simulink model "SolderingIronPIDControllerV2"  (R2024b)
settings: Solver=VariableStepAuto  StartTime=0.0  StopTime=200  RelTol=1e-3
libraries: slpidlib x1
settings Model: Creator=ken  LastModifiedBy=ken

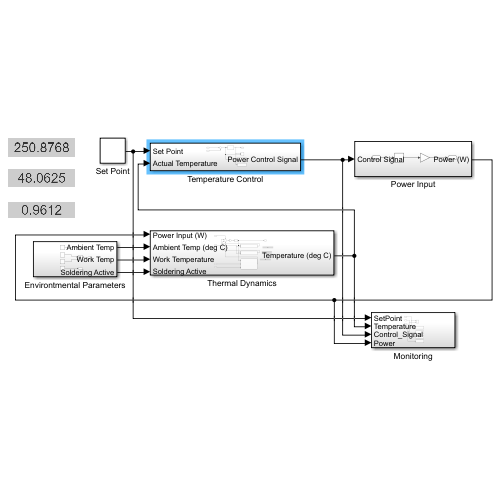
[thumbnail: Simulink's stored preview of the top-level diagram]
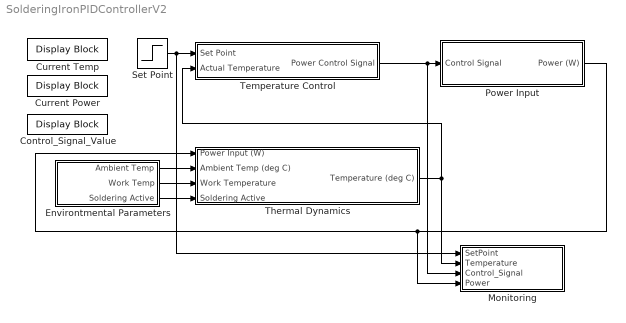
== system SolderingIronPIDControllerV2 ==
  Control_Signal_Value : DisplayBlock  LabelPosition=Hide  Transparency=1
  Current Power : DisplayBlock  LabelPosition=Hide  Transparency=1
  Current Temp : DisplayBlock  LabelPosition=Hide  Transparency=1
  Environtmental Parameters : Subsystem
  Monitoring : Subsystem
  Power Input : Subsystem
  Set Point : Step  Before=250  After=250  SampleTime=0
  Temperature Control : Subsystem
  Thermal Dynamics : Subsystem
  wires:
  Set Point/1 -> Temperature Control/1(Set Point), Monitoring/1(SetPoint)
  Thermal Dynamics/1(Temperature (deg C)) -> Monitoring/2(Temperature), Temperature Control/2(Actual Temperature)
  Temperature Control/1(Power Control Signal) -> Monitoring/3(Control_Signal), Power Input/1(Control Signal)
  Power Input/1(Power (W)) -> Monitoring/4(Power), Thermal Dynamics/1(Power Input (W))
  Environtmental Parameters/1(Ambient Temp) -> Thermal Dynamics/2(Ambient Temp (deg C))
  Environtmental Parameters/2(Work Temp) -> Thermal Dynamics/3(Work Temperature)
  Environtmental Parameters/3(Soldering Active) -> Thermal Dynamics/4(Soldering Active)

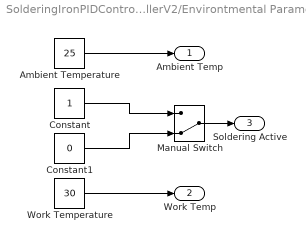
== system SolderingIronPIDControllerV2/Environtmental Parameters ==
  Ambient Temperature : Constant  Value=25
  Constant : Constant
  Constant1 : Constant  Value=0
  Manual Switch : ManualSwitch  CurrentSetting=0
  Work Temperature : Constant  Value=30
  Ambient Temp : Outport
  Work Temp : Outport  Port=2
  Soldering Active : Outport  Port=3
  wires:
  Ambient Temperature/1 -> Ambient Temp/1
  Work Temperature/1 -> Work Temp/1
  Constant/1 -> Manual Switch/1
  Constant1/1 -> Manual Switch/2
  Manual Switch/1 -> Soldering Active/1

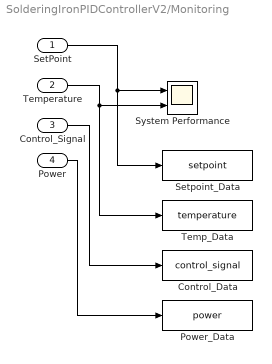
== system SolderingIronPIDControllerV2/Monitoring ==
  SetPoint : Inport
  Temperature : Inport  Port=2
  Control_Signal : Inport  Port=3
  Power : Inport  Port=4
  Control_Data : ToWorkspace  VariableName=control_signal  SaveFormat=Structure With Time  SampleTime=-1
  Power_Data : ToWorkspace  VariableName=power  SaveFormat=Structure With Time  SampleTime=-1
  Setpoint_Data : ToWorkspace  VariableName=setpoint  SaveFormat=Structure With Time  SampleTime=-1
  System Performance : Scope  NumInputPorts=2
  Temp_Data : ToWorkspace  VariableName=temperature  SaveFormat=Structure With Time  SampleTime=-1
  wires:
  SetPoint/1 -> System Performance/1, Setpoint_Data/1
  Temperature/1 -> System Performance/2, Temp_Data/1
  Control_Signal/1 -> Control_Data/1
  Power/1 -> Power_Data/1

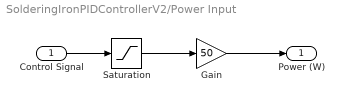
== system SolderingIronPIDControllerV2/Power Input ==
  Control Signal : Inport
  Gain : Gain  Gain=50  OutMax=60
  Saturation : Saturate  UpperLimit=1  LowerLimit=0
  Power (W) : Outport
  wires:
  Control Signal/1 -> Saturation/1
  Saturation/1 -> Gain/1
  Gain/1 -> Power (W)/1

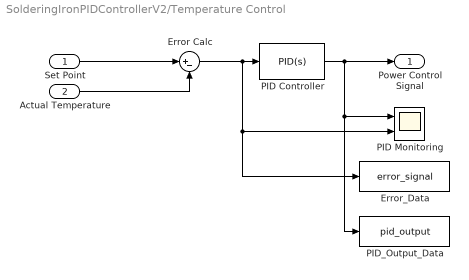
== system SolderingIronPIDControllerV2/Temperature Control ==
  Set Point : Inport
  Actual Temperature : Inport  Port=2
  Error Calc : Sum  Inputs=|+-
  Error_Data : ToWorkspace  VariableName=error_signal  SaveFormat=Structure With Time  SampleTime=-1
  PID Controller : slpidlib/PID Controller  Controller=PID  Form=Parallel  TimeDomain=Continuous-time  UseExternalTs=off  SampleTime=-1  IntegratorMethod=Forward Euler  FilterMethod=Forward Euler  ControllerParametersSource=internal  P=6  I=0.001  UseKiTs=off  D=0.001  UseExternalDerivativeSource=off  N=100  UseFilter=on  TunerSelectOption=Transfer Function Based (PID Tuner App)  InitialConditionSource=internal  InitialConditionForIntegrator=0  InitialConditionForFilter=0  DifferentiatorICPrevScaledInput=0  ExternalReset=none  TrackingMode=off  Kt=1  LimitOutput=on  SatLimitsSource=internal  UpperSaturationLimit=1  LowerSaturationLimit=0  LinearizeAsGain=on  AntiWindupMode=none  Kb=1  LimitIntegrator=off  UpperIntegratorSaturationLimit=inf  LowerIntegratorSaturationLimit=-inf  POutMin=[]  POutMax=[]  IOutMin=[]  IOutMax=[]  DOutMin=[]  DOutMax=[]  NOutMin=[]  NOutMax=[]  SumOutMin=[]  SumOutMax=[]  SaturationOutMin=[]  SaturationOutMax=[]  PParamMin=[]  PParamMax=[]  IParamMin=[]  IParamMax=[]  DParamMin=[]  DParamMax=[]  NParamMin=[]  NParamMax=[]  KbParamMin=[]  KbParamMax=[]  KtParamMin=[]  KtParamMax=[]  KbOutMin=[]  KbOutMax=[]  KtOutMin=[]  KtOutMax=[]  IntegratorOutMin=[]  IntegratorOutMax=[]  FilterOutMin=[]  FilterOutMax=[]  SumI1OutMin=[]  SumI1OutMax=[]  SumI2OutMin=[]  SumI2OutMax=[]  SumI3OutMin=[]  SumI3OutMax=[]  SumI4OutMin=[]  SumI4OutMax=[]  SumDOutMin=[]  SumDOutMax=[]  DifferentiatorOutMin=[]  DifferentiatorOutMax=[]  FilterDiffOutCoefMin=[]  FilterDiffOutCoefMax=[]  ReciprocalOutMin=[]  ReciprocalOutMax=[]  SumDenOutMin=[]  SumDenOutMax=[]  SumNumOutMin=[]  SumNumOutMax=[]  DivideOutMin=[]  DivideOutMax=[]  UdiffTsProdOutMin=[]  UdiffTsProdOutMax=[]  NTsProdOutMin=[]  NTsProdOutMax=[]  UintegralTsProdOutMin=[]  UintegralTsProdOutMax=[]  UngainTsProdOutMin=[]  UngainTsProdOutMax=[]  ClampingZeroOutDataTypeStr=Inherit: Inherit via back propagation  ClampingZeroOutMin=[]  ClampingZeroOutMax=[]  FilterDenConstantOutDataTypeStr=Inherit: Inherit via back propagation  FilterDenConstantOutMin=[]  FilterDenConstantOutMax=[]  PCopyOutDataTypeStr=Inherit: Inherit via back propagation  PCopyOutMin=[]  PCopyOutMax=[]  NCopyOutDataTypeStr=Inherit: Inherit via back propagation  NCopyOutMin=[]  NCopyOutMax=[]  IntegratorContinuousStateAttributes=''  IntegratorStateMustResolveToSignalObject=off  IntegratorRTWStateStorageClass=Auto  FilterContinuousStateAttributes=''  FilterStateMustResolveToSignalObject=off  FilterRTWStateStorageClass=Auto  ParallelPVariant=InternalParameters  IdealPVariant=Disabled  IVariant=InternalParameters  DVariant=InternalParameters  IntegratorVariant=Continuous  SatVariant=Enabled  AWVariant=Passthrough  PCopyVariant=Disabled  TRVariant=Disabled  FdbkBlocksVariant=Forward  IdealPFdbkVariant=Disabled  SatFdbkVariant=Disabled  DerivativeFilterVariant=ContFilter  NVariant=InternalParameters  NCopyVariant=Disabled  FilterICVariant=InternalICsFilter  IntegratorICVariant=InternalICs  ExternalResetVariant=Disabled  TRSumVariant=Passthrough  SumFdbkVariant=Disabled  SumVariant=Sum_PID  TsampFilterVariant=InternalTs  TsampNgainVariant=Passthrough  TsampIntegralVariant=Disabled_SignalSpec  ExternalSaturationOutDataTypeStr=Inherit: Same as second input  DerivativeSourceVariant=ErrorSignal  PreIntVariant=InternalPreInt
  PID Monitoring : Scope  NumInputPorts=2
  PID_Output_Data : ToWorkspace  VariableName=pid_output  SaveFormat=Structure With Time  SampleTime=-1
  Power Control Signal : Outport
  wires:
  Actual Temperature/1 -> Error Calc/2
  Error Calc/1 -> PID Controller/1, PID Monitoring/2, Error_Data/1
  PID Controller/1 -> PID Monitoring/1, PID_Output_Data/1, Power Control Signal/1
  Set Point/1 -> Error Calc/1

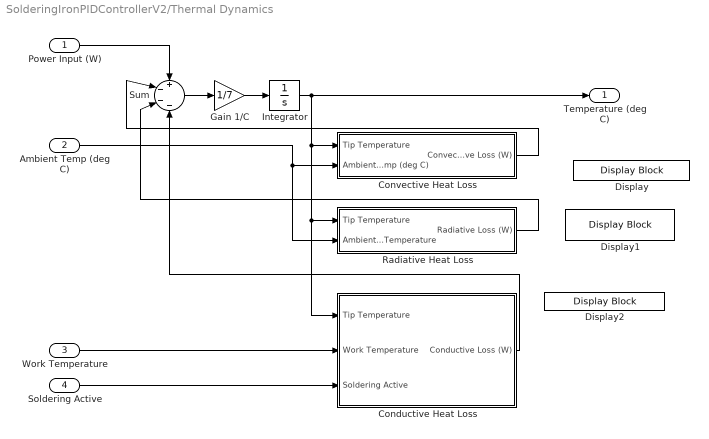
== system SolderingIronPIDControllerV2/Thermal Dynamics ==
  Power Input (W) : Inport
  Ambient Temp (deg C) : Inport  Port=2
  Work Temperature : Inport  Port=3
  Soldering Active : Inport  Port=4
  Conductive Heat Loss : Subsystem
  Convective Heat Loss : Subsystem
  Display : DisplayBlock  LabelPosition=Hide  Transparency=1
  Display1 : DisplayBlock  LabelPosition=Hide  Transparency=1
  Display2 : DisplayBlock  LabelPosition=Hide  Transparency=1
  Gain 1/C : Gain  Gain=1/7
  Integrator : Integrator  InitialCondition=25  LimitOutput=on  UpperSaturationLimit=500  LowerSaturationLimit=25
  Radiative Heat Loss : Subsystem
  Sum : Sum  Inputs=+---
  Temperature (deg C) : Outport
  wires:
  Sum/1 -> Gain 1/C/1
  Gain 1/C/1 -> Integrator/1
  Integrator/1 -> Convective Heat Loss/1(Tip Temperature), Radiative Heat Loss/1(Tip Temperature), Conductive Heat Loss/1(Tip Temperature), Temperature (deg C)/1
  Ambient Temp (deg C)/1 -> Radiative Heat Loss/2(Ambient Temperature), Convective Heat Loss/2(Ambient Temp (deg C))
  Power Input (W)/1 -> Sum/1
  Convective Heat Loss/1(Convective Loss (W)) -> Sum/2
  Radiative Heat Loss/1(Radiative Loss (W)) -> Sum/3
  Conductive Heat Loss/1(Conductive Loss (W)) -> Sum/4
  Soldering Active/1 -> Conductive Heat Loss/3(Soldering Active)
  Work Temperature/1 -> Conductive Heat Loss/2(Work Temperature)

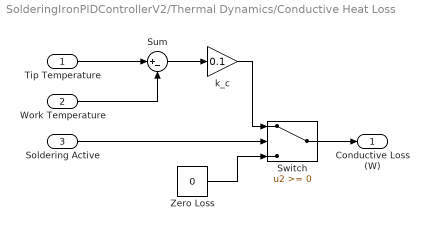
== system SolderingIronPIDControllerV2/Thermal Dynamics/Conductive Heat Loss ==
  Tip Temperature : Inport
  Work Temperature : Inport  Port=2
  Soldering Active : Inport  Port=3
  Sum : Sum  Inputs=|+-
  Switch : Switch  SaturateOnIntegerOverflow=off  InputSameDT=off
  Zero Loss : Constant  Value=0
  k_c : Gain  Gain=0.1
  Conductive Loss (W) : Outport
  wires:
  Tip Temperature/1 -> Sum/1
  Work Temperature/1 -> Sum/2
  Sum/1 -> k_c/1
  k_c/1 -> Switch/1
  Zero Loss/1 -> Switch/3
  Soldering Active/1 -> Switch/2
  Switch/1 -> Conductive Loss (W)/1

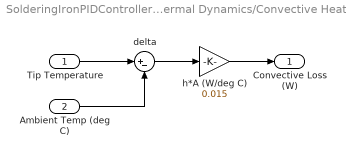
== system SolderingIronPIDControllerV2/Thermal Dynamics/Convective Heat Loss ==
  Tip Temperature : Inport
  Ambient Temp (deg C) : Inport  Port=2
  delta : Sum  Inputs=|+-
  h*A (W/deg C) : Gain  Gain=0.015
  Convective Loss (W) : Outport
  wires:
  Ambient Temp (deg C)/1 -> delta/2
  delta/1 -> h*A (W/deg C)/1
  Tip Temperature/1 -> delta/1
  h*A (W/deg C)/1 -> Convective Loss (W)/1

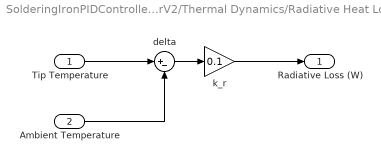
== system SolderingIronPIDControllerV2/Thermal Dynamics/Radiative Heat Loss ==
  Tip Temperature : Inport
  Ambient Temperature : Inport  Port=2
  delta : Sum  Inputs=|+-
  k_r : Gain  Gain=0.1
  Radiative Loss (W) : Outport
  wires:
  Tip Temperature/1 -> delta/1
  Ambient Temperature/1 -> delta/2
  delta/1 -> k_r/1
  k_r/1 -> Radiative Loss (W)/1
